simulink model "SCo1"  (Simulink 8.5)
settings: Solver=ode23tb  SolverMode=SingleTasking  StartTime=0.0  StopTime=0.1  MaxStep=2e-4  RelTol=1e-3  AbsTol=1e-6
libraries: powerlib x81, powerlib_extras x30
settings Model: Creator=azadpour  LastModifiedBy=PC  ExtModeTrigMode=oneshot  ExtModeArmWhenConnect=off
settings DataIOCC: LimitDataPoints=off
settings OptimizationCC: BlockReduction=off  BooleanDataType=off  InitFltsAndDblsToZero=on
settings DebuggingCC: SaveWithParameterizedLinksMsg=none  SignalResolutionControl=TryResolveAllWithWarning  MultiTaskDSMMsg=warning  MultiTaskCondExecSysMsg=none  FcnCallInpInsideContextMsg=UseLocalSettings
settings HardwareCC: TargetUnknown=on
settings GRTTargetCC: TargetFcnLib=ansi_tfl_tmw.mat

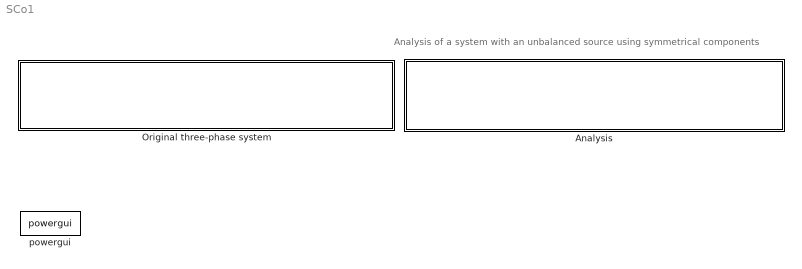
== system SCo1 ==
  note: Analysis of a system with an unbalanced source using symmetrical components
  Analysis : Subsystem
      mask Display: disp('Analysis of the system using Symmetrical Networks');
  Original three-phase system : Subsystem  mask(Original Three-phase system with unbalanced source){}
      mask Display: disp('Original Three-phase system with unbalanced source')
  powergui : powerlib/powergui  SimulationMode=Continuous  SolverType=Tustin/Backward Euler (TBE)  SampleTime=0  frequency=60  SPID=off  DisableSnubberDevices=off  DisableRonSwitches=off  DisableVfSwitches=off  SwTol=0  DisplayEquations=off  Interpol=off  methode=off  Ts=0  FunctionMessages=off  echomessages=off  HookPort=off  EnableUseOfTLC=off  x0status=blocks  frequencyindice=60  Pbase=100e6  ErrMax=1e-4  Iterations=50  UnitsV=kV  UnitsW=MW  buscounter=0  RestoreLinks=warning  ResistiveCurrentMeasurement=off  Frange=[0:2:500]  Ylog=off  Xlog=on  ShowGrid=off  save=off  variable=ZData  structure=0  ZoomFFT=on  StartTime=0.0  cycles=1  DisplayStyle=1  fundamental=60  FreqAxis=off  MaxFrequency=1000  frequencyindicesteady=1  RmsSteady=1  display=off

== system SCo1/Analysis ==
  note: Analysis using symmetrical networks
  Connected Sequence Networks : Subsystem
      mask Display: disp('Connected\n Sequence\n Networks')
  Negative Sequence Network : Subsystem
      mask Display: disp('Negative sequence network')
  Network with source decomposed in  symmetrical components : Subsystem
      mask Display: disp('Network with \nsource decomposed in\n symmetrical components')
  Positive Sequence Network : Subsystem
      mask Display: disp('Positive sequence network')
  Zero Sequence Network : Subsystem
      mask Display: disp('Zero sequence network')

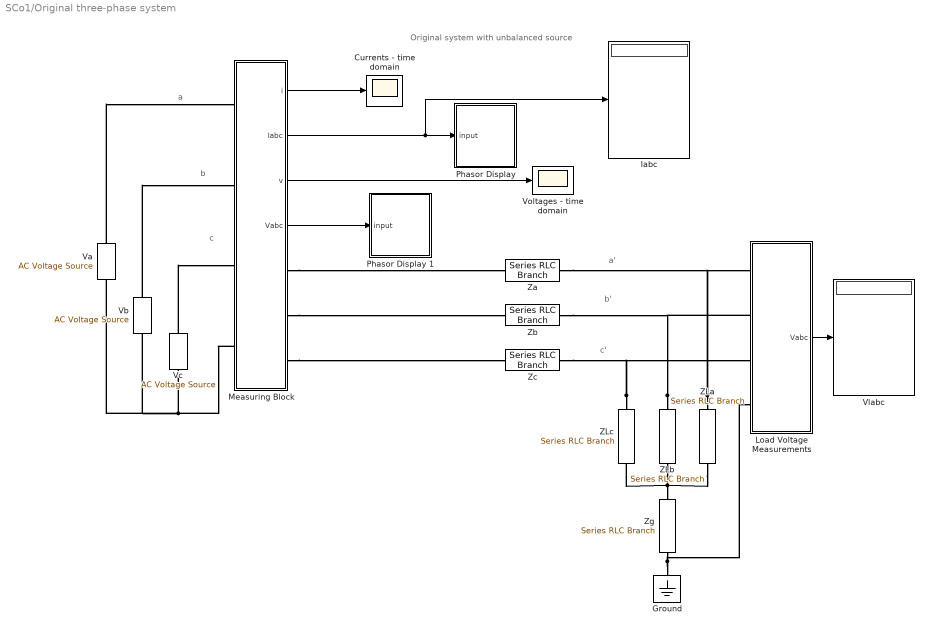
== system SCo1/Original three-phase system ==
  note: a
  note: a'
  note: b
  note: b'
  note: c'
  note: c
  note: Original system with unbalanced source
  Currents - time domain : Scope
      settings: TickLabels=on
  Ground : powerlib/Elements/Ground  LConnTagsString=a
  Iabc : Display
  Load Voltage Measurements : Subsystem
  Measuring Block : Subsystem
  Phasor Display : Subsystem  mask(ABC and 012 Phasor Display){Bactive=off}
      mask prompts: Bactive "Block active"
      mask init:
      | global count;
      | count=0;
      mask Help: web(['file:///' which('uc.html')]);
      mask Display: disp('Display \nabc \nand \n012\nphasors');
  Phasor Display 1 : Subsystem  mask(ABC and 012 Phasor Display){Bactive=off}
      mask prompts: Bactive "Block active"
      mask init:
      | global count;
      | count=0;
      mask Help: web(['file:///' which('uc.html')]);
      mask Display: disp('Display \nabc \nand \n012\nphasors');
  Va : powerlib/Electrical Sources/AC Voltage Source  Amplitude=1  Phase=0  Frequency=60  SampleTime=0  Measurements=None
  Vb : powerlib/Electrical Sources/AC Voltage Source  Amplitude=0.8  Phase=-110  Frequency=60  SampleTime=0  Measurements=None
  Vc : powerlib/Electrical Sources/AC Voltage Source  Amplitude=1.1  Phase=160  Frequency=60  SampleTime=0  Measurements=None
  Vlabc : Display
  Voltages - time domain : Scope
      settings: TickLabels=on
  ZLa : powerlib/Elements/Series RLC Branch  LConnTagsString=__new0  RConnTagsString=__new0  BranchType=RL  Resistance=0.1736  Inductance=0.9848/(2*pi*60)  SetiL0=off  InitialCurrent=0  Capacitance=1.0  Setx0=off  InitialVoltage=0  Measurements=None
  ZLb : powerlib/Elements/Series RLC Branch  LConnTagsString=__new0  RConnTagsString=__new0  BranchType=RL  Resistance=0.1736  Inductance=0.9848/(2*pi*60)  SetiL0=off  InitialCurrent=0  Capacitance=1.0  Setx0=off  InitialVoltage=0  Measurements=None
  ZLc : powerlib/Elements/Series RLC Branch  LConnTagsString=__new0  RConnTagsString=__new0  BranchType=RL  Resistance=0.1736  Inductance=0.9848/(2*pi*60)  SetiL0=off  InitialCurrent=0  Capacitance=1.0  Setx0=off  InitialVoltage=0  Measurements=None
  Za : powerlib/Elements/Series RLC Branch  LConnTagsString=__new0  RConnTagsString=__new0  BranchType=RL  Resistance=0.0347  Inductance=0.1970/(2*pi*60)  SetiL0=off  InitialCurrent=0  Capacitance=1.0  Setx0=off  InitialVoltage=0  Measurements=None
  Zb : powerlib/Elements/Series RLC Branch  LConnTagsString=__new0  RConnTagsString=__new0  BranchType=RL  Resistance=0.0347  Inductance=0.1970/(2*pi*60)  SetiL0=off  InitialCurrent=0  Capacitance=1.0  Setx0=off  InitialVoltage=0  Measurements=None
  Zc : powerlib/Elements/Series RLC Branch  LConnTagsString=__new0  RConnTagsString=__new0  BranchType=RL  Resistance=0.0347  Inductance=0.1970/(2*pi*60)  SetiL0=off  InitialCurrent=0  Capacitance=1.0  Setx0=off  InitialVoltage=0  Measurements=None
  Zg : powerlib/Elements/Series RLC Branch  LConnTagsString=__new0  RConnTagsString=__new0  BranchType=RL  Resistance=0.0695  Inductance=0.3939/(2*pi*60)  SetiL0=off  InitialCurrent=0  Capacitance=1.0  Setx0=off  InitialVoltage=0  Measurements=None
  wires:
  Measuring Block/1(i) -> Currents - time domain/1
  Measuring Block/3(v) -> Voltages - time domain/1
  Measuring Block/4(Vabc) -> Phasor Display 1/1(input)
  Load Voltage Measurements/1(Vabc) -> Vlabc/1
  Measuring Block/2(Iabc) -> Phasor Display/1(input), Iabc/1
  connections:
  Measuring Block/RConn1 -- Za/LConn1
  Measuring Block/RConn2 -- Zb/LConn1
  Measuring Block/RConn3 -- Zc/LConn1
  Va/LConn1 -- Vb/LConn1 -- Measuring Block/LConn4 -- Vc/LConn1
  Va/RConn1 -- Measuring Block/LConn1
  Vb/RConn1 -- Measuring Block/LConn2
  Vc/RConn1 -- Measuring Block/LConn3
  ZLb/RConn1 -- ZLa/RConn1 -- ZLc/RConn1 -- Zg/LConn1
  ZLb/LConn1 -- Load Voltage Measurements/LConn2 -- Zb/RConn1
  Ground/LConn1 -- Load Voltage Measurements/LConn4 -- Zg/RConn1
  ZLc/LConn1 -- Zc/RConn1 -- Load Voltage Measurements/LConn3
  ZLa/LConn1 -- Za/RConn1 -- Load Voltage Measurements/LConn1

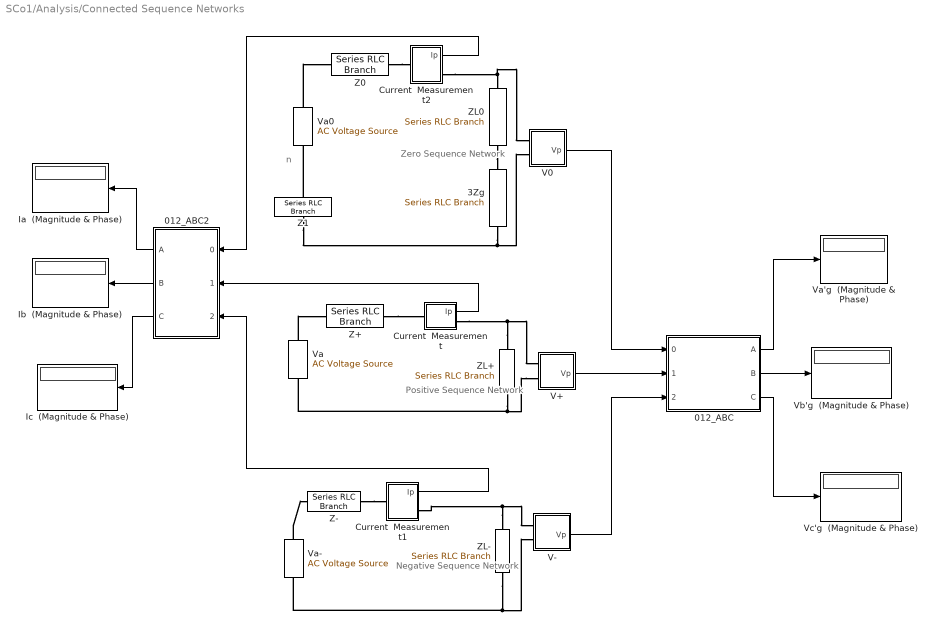
== system SCo1/Analysis/Connected Sequence Networks ==
  note: Positive Sequence Network
  note: Negative Sequence Network
  note: Zero Sequence Network
  note: n
  012_ABC : Subsystem
      mask init:
      | a=cos(120*pi/180)+i*sin(120*pi/180);
      | A=[1 1 1; 1 a^2 a; 1 a a^2];
      mask Display: disp('012_ABC');
  012_ABC2 : Subsystem
      mask init:
      | a=cos(120*pi/180)+i*sin(120*pi/180);
      | A=[1 1 1; 1 a^2 a; 1 a a^2];
      mask Display: disp('012_ABC');
  3Zg : powerlib/Elements/Series RLC Branch  LConnTagsString=__new0  RConnTagsString=__new0  BranchType=RL  Resistance=3*0.0695  Inductance=3*0.3939/(2*pi*60)  SetiL0=off  InitialCurrent=0  Capacitance=1.0  Setx0=off  InitialVoltage=0  Measurements=None
  Current  Measurement : Subsystem
  Current  Measurement1 : Subsystem
  Current  Measurement2 : Subsystem
  Ia  (Magnitude & Phase) : Display
  Ib  (Magnitude & Phase) : Display
  Ic  (Magnitude & Phase) : Display
  V+ : Subsystem
  V- : Subsystem
  V0 : Subsystem
  Va : powerlib/Electrical Sources/AC Voltage Source  Amplitude=0.92  Phase=17.8  Frequency=60  SampleTime=0  Measurements=None
  Va'g  (Magnitude & Phase) : Display
  Va- : powerlib/Electrical Sources/AC Voltage Source  Amplitude=0.27  Phase=-34.8  Frequency=60  SampleTime=0  Measurements=None
  Va0 : powerlib/Electrical Sources/AC Voltage Source  Amplitude=0.16  Phase=-129.3  Frequency=60  SampleTime=0  Measurements=None
  Vb'g  (Magnitude & Phase) : Display
  Vc'g  (Magnitude & Phase) : Display
  Z+ : powerlib/Elements/Series RLC Branch  LConnTagsString=__new0  RConnTagsString=__new0  BranchType=RL  Resistance=0.0347  Inductance=0.1970/(2*pi*60)  SetiL0=off  InitialCurrent=0  Capacitance=1.0  Setx0=off  InitialVoltage=0  Measurements=None
  Z- : powerlib/Elements/Series RLC Branch  LConnTagsString=__new0  RConnTagsString=__new0  BranchType=RL  Resistance=0.0347  Inductance=0.1970/(2*pi*60)  SetiL0=off  InitialCurrent=0  Capacitance=1.0  Setx0=off  InitialVoltage=0  Measurements=None
  Z0 : powerlib/Elements/Series RLC Branch  LConnTagsString=__new0  RConnTagsString=__new0  BranchType=RL  Resistance=0.0347  Inductance=0.1970/(2*pi*60)  SetiL0=off  InitialCurrent=0  Capacitance=1.0  Setx0=off  InitialVoltage=0  Measurements=None
  Z1 : powerlib/Elements/Series RLC Branch  LConnTagsString=__new0  RConnTagsString=__new0  BranchType=R  Resistance=1e10  Inductance=1.0  SetiL0=off  InitialCurrent=0  Capacitance=1.0  Setx0=off  InitialVoltage=0  Measurements=None
  ZL+ : powerlib/Elements/Series RLC Branch  LConnTagsString=__new0  RConnTagsString=__new0  BranchType=RL  Resistance=0.1736  Inductance=0.9848/(2*pi*60)  SetiL0=off  InitialCurrent=0  Capacitance=1.0  Setx0=off  InitialVoltage=0  Measurements=None
  ZL- : powerlib/Elements/Series RLC Branch  LConnTagsString=__new0  RConnTagsString=__new0  BranchType=RL  Resistance=0.1736  Inductance=0.9848/(2*pi*60)  SetiL0=off  InitialCurrent=0  Capacitance=1.0  Setx0=off  InitialVoltage=0  Measurements=None
  ZL0 : powerlib/Elements/Series RLC Branch  LConnTagsString=__new0  RConnTagsString=__new0  BranchType=RL  Resistance=0.1736  Inductance=0.9848/(2*pi*60)  SetiL0=off  InitialCurrent=0  Capacitance=1.0  Setx0=off  InitialVoltage=0  Measurements=None
  wires:
  012_ABC/1(A) -> Va'g  (Magnitude & Phase)/1
  012_ABC/2(B) -> Vb'g  (Magnitude & Phase)/1
  012_ABC/3(C) -> Vc'g  (Magnitude & Phase)/1
  012_ABC2/1(A) -> Ia  (Magnitude & Phase)/1
  012_ABC2/2(B) -> Ib  (Magnitude & Phase)/1
  012_ABC2/3(C) -> Ic  (Magnitude & Phase)/1
  Current  Measurement/1(Ip) -> 012_ABC2/2(1)
  V+/1(Vp) -> 012_ABC/2(1)
  V-/1(Vp) -> 012_ABC/3(2)
  Current  Measurement1/1(Ip) -> 012_ABC2/3(2)
  V0/1(Vp) -> 012_ABC/1(0)
  Current  Measurement2/1(Ip) -> 012_ABC2/1(0)
  connections:
  V+/LConn2 -- Va/LConn1 -- ZL+/RConn1
  ZL+/LConn1 -- Current  Measurement/RConn1 -- V+/LConn1
  Va-/LConn1 -- ZL-/RConn1 -- V-/LConn2
  ZL-/LConn1 -- Current  Measurement1/RConn1 -- V-/LConn1
  ZL0/LConn1 -- Current  Measurement2/RConn1 -- V0/LConn1
  3Zg/RConn1 -- Z1/LConn1 -- V0/LConn2
  Z+/RConn1 -- Current  Measurement/LConn1
  Z-/RConn1 -- Current  Measurement1/LConn1
  Va-/RConn1 -- Z-/LConn1
  Z0/RConn1 -- Current  Measurement2/LConn1
  Z1/RConn1 -- Va0/LConn1
  Va0/RConn1 -- Z0/LConn1
  Va/RConn1 -- Z+/LConn1
  ZL0/RConn1 -- 3Zg/LConn1

== system SCo1/Analysis/Negative Sequence Network ==
  Current  Measurement : Subsystem
  "Ia- (Magnitude & Phase) " : Display
  V- : Subsystem
  Va'g- (Magnitude & Phase) : Display
  Va- : powerlib/Electrical Sources/AC Voltage Source  Amplitude=0.27  Phase=-34.8  Frequency=60  SampleTime=0  Measurements=None
  ZLa : powerlib/Elements/Series RLC Branch  LConnTagsString=__new0  RConnTagsString=__new0  BranchType=RL  Resistance=0.1736  Inductance=0.9848/(2*pi*60)  SetiL0=off  InitialCurrent=0  Capacitance=1.0  Setx0=off  InitialVoltage=0  Measurements=None
  Za : powerlib/Elements/Series RLC Branch  LConnTagsString=__new0  RConnTagsString=__new0  BranchType=RL  Resistance=0.0347  Inductance=0.1970/(2*pi*60)  SetiL0=off  InitialCurrent=0  Capacitance=1.0  Setx0=off  InitialVoltage=0  Measurements=None
  wires:
  Current  Measurement/1(Ip) -> "Ia- (Magnitude & Phase) "/1
  V-/1(V) -> Va'g- (Magnitude & Phase)/1
  connections:
  Va-/RConn1 -- Za/LConn1
  ZLa/RConn1 -- V-/LConn2 -- Va-/LConn1
  Za/RConn1 -- Current  Measurement/LConn1
  Current  Measurement/RConn1 -- V-/LConn1 -- ZLa/LConn1

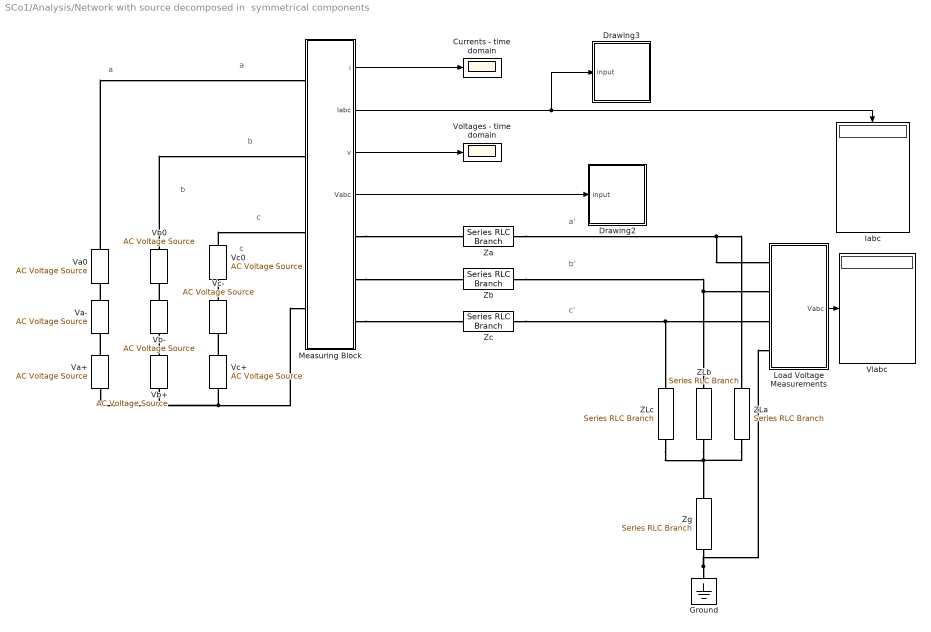
== system SCo1/Analysis/Network with source decomposed in  symmetrical components ==
  note: a
  note: b
  note: a
  note: a'
  note: b
  note: b'
  note: c'
  note: c
  note: c
  Currents - time domain : Scope
      settings: TickLabels=on
  Drawing2 : Subsystem  mask(ABC and 012 Phasor Display){Bactive=off}
      mask prompts: Bactive "Block active"
      mask init:
      | global count;
      | count=0;
      mask Help: web(['file:///' which('uc.html')]);
      mask Display: disp('Display \nabc \nand \n012\nphasors');
  Drawing3 : Subsystem  mask(ABC and 012 Phasor Display){Bactive=off}
      mask prompts: Bactive "Block active"
      mask init:
      | global count;
      | count=0;
      mask Help: web(['file:///' which('uc.html')]);
      mask Display: disp('Display \nabc \nand \n012\nphasors');
  Ground : powerlib/Elements/Ground  LConnTagsString=a
  Iabc : Display
  Load Voltage Measurements : Subsystem
  Measuring Block : Subsystem
  Va+ : powerlib/Electrical Sources/AC Voltage Source  Amplitude=0.92  Phase=17.8  Frequency=60  SampleTime=0  Measurements=None
  Va- : powerlib/Electrical Sources/AC Voltage Source  Amplitude=0.27  Phase=-34.8  Frequency=60  SampleTime=0  Measurements=None
  Va0 : powerlib/Electrical Sources/AC Voltage Source  Amplitude=0.16  Phase=-129.3  Frequency=60  SampleTime=0  Measurements=None
  Vb+ : powerlib/Electrical Sources/AC Voltage Source  Amplitude=0.92  Phase=17.8-120  Frequency=60  SampleTime=0  Measurements=None
  Vb- : powerlib/Electrical Sources/AC Voltage Source  Amplitude=0.27  Phase=-34.8+120  Frequency=60  SampleTime=0  Measurements=None
  Vb0 : powerlib/Electrical Sources/AC Voltage Source  Amplitude=0.16  Phase=-129.3  Frequency=60  SampleTime=0  Measurements=None
  Vc+ : powerlib/Electrical Sources/AC Voltage Source  Amplitude=0.92  Phase=17.8+120  Frequency=60  SampleTime=0  Measurements=None
  Vc- : powerlib/Electrical Sources/AC Voltage Source  Amplitude=0.27  Phase=-34.8-120  Frequency=60  SampleTime=0  Measurements=None
  Vc0 : powerlib/Electrical Sources/AC Voltage Source  Amplitude=0.16  Phase=-129.3  Frequency=60  SampleTime=0  Measurements=None
  Vlabc : Display
  Voltages - time domain : Scope
      settings: TickLabels=on
  ZLa : powerlib/Elements/Series RLC Branch  LConnTagsString=__new0  RConnTagsString=__new0  BranchType=RL  Resistance=0.1736  Inductance=0.9848/(2*pi*60)  SetiL0=off  InitialCurrent=0  Capacitance=1.0  Setx0=off  InitialVoltage=0  Measurements=None
  ZLb : powerlib/Elements/Series RLC Branch  LConnTagsString=__new0  RConnTagsString=__new0  BranchType=RL  Resistance=0.1736  Inductance=0.9848/(2*pi*60)  SetiL0=off  InitialCurrent=0  Capacitance=1.0  Setx0=off  InitialVoltage=0  Measurements=None
  ZLc : powerlib/Elements/Series RLC Branch  LConnTagsString=__new0  RConnTagsString=__new0  BranchType=RL  Resistance=0.1736  Inductance=0.9848/(2*pi*60)  SetiL0=off  InitialCurrent=0  Capacitance=1.0  Setx0=off  InitialVoltage=0  Measurements=None
  Za : powerlib/Elements/Series RLC Branch  LConnTagsString=__new0  RConnTagsString=__new0  BranchType=RL  Resistance=0.0347  Inductance=0.1970/(2*pi*60)  SetiL0=off  InitialCurrent=0  Capacitance=1.0  Setx0=off  InitialVoltage=0  Measurements=None
  Zb : powerlib/Elements/Series RLC Branch  LConnTagsString=__new0  RConnTagsString=__new0  BranchType=RL  Resistance=0.0347  Inductance=0.1970/(2*pi*60)  SetiL0=off  InitialCurrent=0  Capacitance=1.0  Setx0=off  InitialVoltage=0  Measurements=None
  Zc : powerlib/Elements/Series RLC Branch  LConnTagsString=__new0  RConnTagsString=__new0  BranchType=RL  Resistance=0.0347  Inductance=0.1970/(2*pi*60)  SetiL0=off  InitialCurrent=0  Capacitance=1.0  Setx0=off  InitialVoltage=0  Measurements=None
  Zg : powerlib/Elements/Series RLC Branch  LConnTagsString=__new0  RConnTagsString=__new0  BranchType=RL  Resistance=0.0695  Inductance=0.3939/(2*pi*60)  SetiL0=off  InitialCurrent=0  Capacitance=1.0  Setx0=off  InitialVoltage=0  Measurements=None
  wires:
  Load Voltage Measurements/1(Vabc) -> Vlabc/1
  Measuring Block/1(i) -> Currents - time domain/1
  Measuring Block/3(v) -> Voltages - time domain/1
  Measuring Block/4(Vabc) -> Drawing2/1(input)
  Measuring Block/2(Iabc) -> Iabc/1, Drawing3/1(input)
  connections:
  Measuring Block/RConn1 -- Za/LConn1
  Measuring Block/RConn2 -- Zb/LConn1
  Measuring Block/RConn3 -- Zc/LConn1
  Vb0/RConn1 -- Measuring Block/LConn2
  Va0/RConn1 -- Measuring Block/LConn1
  Vc0/RConn1 -- Measuring Block/LConn3
  Va-/RConn1 -- Va0/LConn1
  Ground/LConn1 -- Load Voltage Measurements/LConn4 -- Zg/RConn1
  Zc/RConn1 -- ZLc/LConn1 -- Load Voltage Measurements/LConn3
  Zb/RConn1 -- ZLb/LConn1 -- Load Voltage Measurements/LConn2
  Za/RConn1 -- ZLa/LConn1 -- Load Voltage Measurements/LConn1
  Va+/RConn1 -- Va-/LConn1
  Vb+/RConn1 -- Vb-/LConn1
  Vc+/RConn1 -- Vc-/LConn1
  Vc-/RConn1 -- Vc0/LConn1
  Vb-/RConn1 -- Vb0/LConn1
  Va+/LConn1 -- Vb+/LConn1 -- Measuring Block/LConn4 -- Vc+/LConn1
  ZLb/RConn1 -- Zg/LConn1 -- ZLa/RConn1 -- ZLc/RConn1

== system SCo1/Analysis/Positive Sequence Network ==
  Current  Measurement : Subsystem
  Ia+ (Magnitude & Phase)1 : Display
  V+ : Subsystem
  Va'g+ (Magnitude & Phase) : Display
  Va+ : powerlib/Electrical Sources/AC Voltage Source  Amplitude=0.92  Phase=17.8  Frequency=60  SampleTime=0  Measurements=None
  ZLa : powerlib/Elements/Series RLC Branch  LConnTagsString=__new0  RConnTagsString=__new0  BranchType=RL  Resistance=0.1736  Inductance=0.9848/(2*pi*60)  SetiL0=off  InitialCurrent=0  Capacitance=1.0  Setx0=off  InitialVoltage=0  Measurements=None
  Za : powerlib/Elements/Series RLC Branch  LConnTagsString=__new0  RConnTagsString=__new0  BranchType=RL  Resistance=0.0347  Inductance=0.1970/(2*pi*60)  SetiL0=off  InitialCurrent=0  Capacitance=1.0  Setx0=off  InitialVoltage=0  Measurements=None
  wires:
  V+/1(V) -> Va'g+ (Magnitude & Phase)/1
  Current  Measurement/1(Ip) -> Ia+ (Magnitude & Phase)1/1
  connections:
  Va+/RConn1 -- Za/LConn1
  ZLa/RConn1 -- V+/LConn2 -- Va+/LConn1
  Za/RConn1 -- Current  Measurement/LConn1
  Current  Measurement/RConn1 -- ZLa/LConn1 -- V+/LConn1

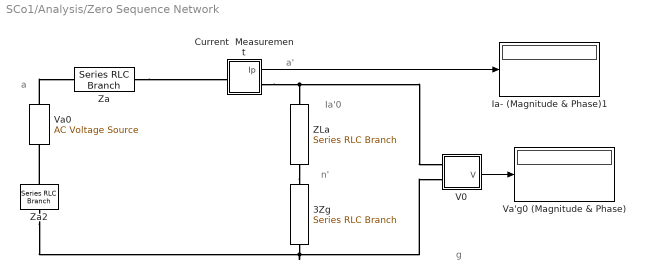
== system SCo1/Analysis/Zero Sequence Network ==
  note: n'
  note: a
  note: a'
  note: g
  note: Ia'0
  3Zg : powerlib/Elements/Series RLC Branch  LConnTagsString=__new0  RConnTagsString=__new0  BranchType=RL  Resistance=3*0.0695  Inductance=3*0.3939/(2*pi*60)  SetiL0=off  InitialCurrent=0  Capacitance=1.0  Setx0=off  InitialVoltage=0  Measurements=None
  Current  Measurement : Subsystem
  Ia- (Magnitude & Phase)1 : Display
      settings: Decimation=2
  V0 : Subsystem
  Va'g0 (Magnitude & Phase) : Display
  Va0 : powerlib/Electrical Sources/AC Voltage Source  Amplitude=0.16  Phase=-129.3  Frequency=60  SampleTime=0  Measurements=None
  ZLa : powerlib/Elements/Series RLC Branch  LConnTagsString=__new0  RConnTagsString=__new0  BranchType=RL  Resistance=0.1736  Inductance=0.9848/(2*pi*60)  SetiL0=off  InitialCurrent=0  Capacitance=1.0  Setx0=off  InitialVoltage=0  Measurements=None
  Za : powerlib/Elements/Series RLC Branch  LConnTagsString=__new0  RConnTagsString=__new0  BranchType=RL  Resistance=0.0347  Inductance=0.1970/(2*pi*60)  SetiL0=off  InitialCurrent=0  Capacitance=1.0  Setx0=off  InitialVoltage=0  Measurements=None
  Za2 : powerlib/Elements/Series RLC Branch  LConnTagsString=__new0  RConnTagsString=__new0  BranchType=Open circuit  Resistance=1  Inductance=1e-3  SetiL0=off  InitialCurrent=0  Capacitance=1e-6  Setx0=off  InitialVoltage=0  Measurements=None
  wires:
  V0/1(V) -> Va'g0 (Magnitude & Phase)/1
  Current  Measurement/1(Ip) -> Ia- (Magnitude & Phase)1/1
  connections:
  ZLa/RConn1 -- 3Zg/LConn1
  Va0/RConn1 -- Za/LConn1
  Za/RConn1 -- Current  Measurement/LConn1
  Za2/RConn1 -- 3Zg/RConn1 -- V0/LConn2
  Current  Measurement/RConn1 -- V0/LConn1 -- ZLa/LConn1
  Za2/LConn1 -- Va0/LConn1

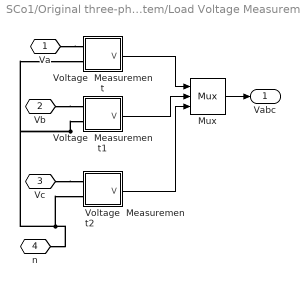
== system SCo1/Original three-phase system/Load Voltage Measurements ==
  Mux : Mux  Inputs=3
  Voltage  Measurement : Subsystem
  Voltage  Measurement1 : Subsystem
  Voltage  Measurement2 : Subsystem
  Va : PMIOPort  Port=1  Side=Left
  Vb : PMIOPort  Port=2  Side=Left
  Vc : PMIOPort  Port=3  Side=Left
  n : PMIOPort  Port=4  Side=Left
  Vabc : Outport  InitialOutput=0
  wires:
  Voltage  Measurement/1(V) -> Mux/1
  Voltage  Measurement1/1(V) -> Mux/2
  Voltage  Measurement2/1(V) -> Mux/3
  Mux/1 -> Vabc/1
  connections:
  Va/RConn1 -- Voltage  Measurement/LConn1
  Vb/RConn1 -- Voltage  Measurement1/LConn1
  Vc/RConn1 -- Voltage  Measurement2/LConn1
  n/RConn1 -- Voltage  Measurement2/LConn2 -- Voltage  Measurement1/LConn2 -- Voltage  Measurement/LConn2

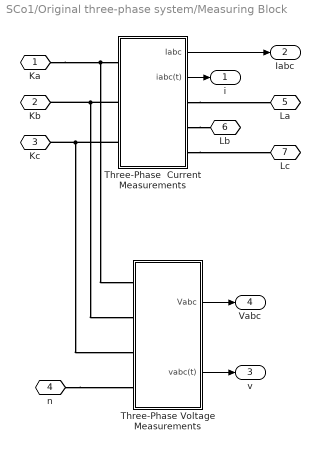
== system SCo1/Original three-phase system/Measuring Block ==
  Three-Phase Voltage Measurements : Subsystem
  Three-Phase  Current Measurements : Subsystem
  Ka : PMIOPort  Port=1  Side=Left
  Kb : PMIOPort  Port=2  Side=Left
  Kc : PMIOPort  Port=3  Side=Left
  n : PMIOPort  Port=4  Side=Left
  La : PMIOPort  Port=5  Side=Right
  Lb : PMIOPort  Port=6  Side=Right
  Lc : PMIOPort  Port=7  Side=Right
  i : Outport
  Iabc : Outport  Port=2
  v : Outport  Port=3
  Vabc : Outport  Port=4
  wires:
  Three-Phase  Current Measurements/1(Iabc) -> Iabc/1
  Three-Phase Voltage Measurements/1(Vabc) -> Vabc/1
  Three-Phase  Current Measurements/2(iabc(t)) -> i/1
  Three-Phase Voltage Measurements/2(vabc(t)) -> v/1
  connections:
  Three-Phase  Current Measurements/RConn3 -- Lc/RConn1
  Three-Phase  Current Measurements/RConn2 -- Lb/RConn1
  Three-Phase  Current Measurements/RConn1 -- La/RConn1
  n/RConn1 -- Three-Phase Voltage Measurements/LConn4
  Ka/RConn1 -- Three-Phase  Current Measurements/LConn1 -- Three-Phase Voltage Measurements/LConn1
  Three-Phase  Current Measurements/LConn2 -- Kb/RConn1 -- Three-Phase Voltage Measurements/LConn2
  Three-Phase  Current Measurements/LConn3 -- Kc/RConn1 -- Three-Phase Voltage Measurements/LConn3

== system SCo1/Original three-phase system/Phasor Display ==
  input : Inport
  S-Function : S-Function  FunctionName=phdraw1c  Parameters=Bactive
  wires:
  input/1 -> S-Function/1

== system SCo1/Original three-phase system/Phasor Display 1 ==
  input : Inport
  S-Function : S-Function  FunctionName=phdraw1c  Parameters=Bactive
  wires:
  input/1 -> S-Function/1

== system SCo1/Analysis/Connected Sequence Networks/012_ABC ==
  0 : Inport
  1 : Inport  Port=2
  2 : Inport  Port=3
  Demux : Demux  Outputs=3
  Mux3 : Mux  Inputs=3
  S-Function : S-Function  FunctionName=pnz_ABC  Parameters=A
  A : Outport  InitialOutput=0
  B : Outport  Port=2  InitialOutput=0
  C : Outport  Port=3  InitialOutput=0
  wires:
  Mux3/1 -> S-Function/1
  0/1 -> Mux3/1
  1/1 -> Mux3/2
  2/1 -> Mux3/3
  S-Function/1 -> Demux/1
  Demux/1 -> A/1
  Demux/2 -> B/1
  Demux/3 -> C/1

== system SCo1/Analysis/Connected Sequence Networks/012_ABC2 ==
  0 : Inport
  1 : Inport  Port=2
  2 : Inport  Port=3
  Demux : Demux  Outputs=3
  Mux3 : Mux  Inputs=3
  S-Function : S-Function  FunctionName=pnz_ABC  Parameters=A
  A : Outport  InitialOutput=0
  B : Outport  Port=2  InitialOutput=0
  C : Outport  Port=3  InitialOutput=0
  wires:
  Demux/3 -> C/1
  Demux/2 -> B/1
  Demux/1 -> A/1
  S-Function/1 -> Demux/1
  2/1 -> Mux3/3
  1/1 -> Mux3/2
  0/1 -> Mux3/1
  Mux3/1 -> S-Function/1

== system SCo1/Analysis/Connected Sequence Networks/Current  Measurement ==
  Current Measurement1 : powerlib/Measurements/Current Measurement  PhasorSimulation=off  OutputType=Magnitude  PSBequivalent=0
  Fourier1 : powerlib_extras/Measurements/Fourier  f1=60  n=1
  Mux1 : Mux  Inputs=2
  + : PMIOPort  Port=1  Side=Left
  - : PMIOPort  Port=2  Side=Right
  Ip : Outport  InitialOutput=0
  wires:
  Fourier1/2 -> Mux1/2
  Fourier1/1 -> Mux1/1
  Mux1/1 -> Ip/1
  Current Measurement1/1 -> Fourier1/1
  connections:
  +/RConn1 -- Current Measurement1/LConn1
  Current Measurement1/RConn1 -- -/RConn1

== system SCo1/Analysis/Connected Sequence Networks/Current  Measurement1 ==
  Current Measurement1 : powerlib/Measurements/Current Measurement  PhasorSimulation=off  OutputType=Magnitude  PSBequivalent=0
  Fourier1 : powerlib_extras/Measurements/Fourier  f1=60  n=1
  Mux1 : Mux  Inputs=2
  + : PMIOPort  Port=1  Side=Left
  - : PMIOPort  Port=2  Side=Right
  Ip : Outport  InitialOutput=0
  wires:
  Fourier1/2 -> Mux1/2
  Fourier1/1 -> Mux1/1
  Mux1/1 -> Ip/1
  Current Measurement1/1 -> Fourier1/1
  connections:
  +/RConn1 -- Current Measurement1/LConn1
  Current Measurement1/RConn1 -- -/RConn1

== system SCo1/Analysis/Connected Sequence Networks/Current  Measurement2 ==
  Current Measurement1 : powerlib/Measurements/Current Measurement  PhasorSimulation=off  OutputType=Magnitude  PSBequivalent=0
  Fourier1 : powerlib_extras/Measurements/Fourier  f1=60  n=1
  Mux1 : Mux  Inputs=2
  + : PMIOPort  Port=1  Side=Left
  - : PMIOPort  Port=2  Side=Right
  Ip : Outport  InitialOutput=0
  wires:
  Fourier1/2 -> Mux1/2
  Fourier1/1 -> Mux1/1
  Mux1/1 -> Ip/1
  Current Measurement1/1 -> Fourier1/1
  connections:
  +/RConn1 -- Current Measurement1/LConn1
  Current Measurement1/RConn1 -- -/RConn1

== system SCo1/Analysis/Connected Sequence Networks/V+ ==
  Fourier2 : powerlib_extras/Measurements/Fourier  f1=60  n=1
  Mux3 : Mux  Inputs=2
  Voltage Measurement1 : powerlib/Measurements/Voltage Measurement  PhasorSimulation=off  OutputType=Magnitude  PSBequivalent=0
  + : PMIOPort  Port=1  Side=Left
  - : PMIOPort  Port=2  Side=Left
  Vp : Outport  InitialOutput=0
  wires:
  Fourier2/1 -> Mux3/1
  Fourier2/2 -> Mux3/2
  Mux3/1 -> Vp/1
  Voltage Measurement1/1 -> Fourier2/1
  connections:
  +/RConn1 -- Voltage Measurement1/LConn1
  -/RConn1 -- Voltage Measurement1/LConn2

== system SCo1/Analysis/Connected Sequence Networks/V- ==
  Fourier2 : powerlib_extras/Measurements/Fourier  f1=60  n=1
  Mux3 : Mux  Inputs=2
  Voltage Measurement1 : powerlib/Measurements/Voltage Measurement  PhasorSimulation=off  OutputType=Magnitude  PSBequivalent=0
  + : PMIOPort  Port=1  Side=Left
  - : PMIOPort  Port=2  Side=Left
  Vp : Outport  InitialOutput=0
  wires:
  Fourier2/1 -> Mux3/1
  Fourier2/2 -> Mux3/2
  Mux3/1 -> Vp/1
  Voltage Measurement1/1 -> Fourier2/1
  connections:
  +/RConn1 -- Voltage Measurement1/LConn1
  -/RConn1 -- Voltage Measurement1/LConn2

== system SCo1/Analysis/Connected Sequence Networks/V0 ==
  Fourier2 : powerlib_extras/Measurements/Fourier  f1=60  n=1
  Mux3 : Mux  Inputs=2
  Voltage Measurement1 : powerlib/Measurements/Voltage Measurement  PhasorSimulation=off  OutputType=Magnitude  PSBequivalent=0
  + : PMIOPort  Port=1  Side=Left
  - : PMIOPort  Port=2  Side=Left
  Vp : Outport  InitialOutput=0
  wires:
  Mux3/1 -> Vp/1
  Fourier2/2 -> Mux3/2
  Fourier2/1 -> Mux3/1
  Voltage Measurement1/1 -> Fourier2/1
  connections:
  -/RConn1 -- Voltage Measurement1/LConn2
  +/RConn1 -- Voltage Measurement1/LConn1

== system SCo1/Analysis/Negative Sequence Network/Current  Measurement ==
  Current Measurement1 : powerlib/Measurements/Current Measurement  PhasorSimulation=off  OutputType=Magnitude  PSBequivalent=0
  Fourier1 : powerlib_extras/Measurements/Fourier  f1=60  n=1
  Mux : Mux  Inputs=2
  + : PMIOPort  Port=1  Side=Left
  - : PMIOPort  Port=2  Side=Right
  Ip : Outport  InitialOutput=0
  wires:
  Fourier1/2 -> Mux/2
  Fourier1/1 -> Mux/1
  Current Measurement1/1 -> Fourier1/1
  Mux/1 -> Ip/1
  connections:
  +/RConn1 -- Current Measurement1/LConn1
  Current Measurement1/RConn1 -- -/RConn1

== system SCo1/Analysis/Negative Sequence Network/V- ==
  Fourier2 : powerlib_extras/Measurements/Fourier  f1=60  n=1
  Mux3 : Mux  Inputs=2
  Voltage Measurement1 : powerlib/Measurements/Voltage Measurement  PhasorSimulation=off  OutputType=Magnitude  PSBequivalent=0
  + : PMIOPort  Port=1  Side=Left
  - : PMIOPort  Port=2  Side=Left
  V : Outport  InitialOutput=0
  wires:
  Fourier2/1 -> Mux3/1
  Fourier2/2 -> Mux3/2
  Mux3/1 -> V/1
  Voltage Measurement1/1 -> Fourier2/1
  connections:
  +/RConn1 -- Voltage Measurement1/LConn1
  -/RConn1 -- Voltage Measurement1/LConn2

== system SCo1/Analysis/Network with source decomposed in  symmetrical components/Drawing2 ==
  input : Inport
  S-Function : S-Function  FunctionName=phdraw1c  Parameters=Bactive
  wires:
  input/1 -> S-Function/1

== system SCo1/Analysis/Network with source decomposed in  symmetrical components/Drawing3 ==
  input : Inport
  S-Function : S-Function  FunctionName=phdraw1c  Parameters=Bactive
  wires:
  input/1 -> S-Function/1

== system SCo1/Analysis/Network with source decomposed in  symmetrical components/Load Voltage Measurements ==
  Mux : Mux  Inputs=3
  Voltage  Measurement : Subsystem
  Voltage  Measurement1 : Subsystem
  Voltage  Measurement2 : Subsystem
  Va : PMIOPort  Port=1  Side=Left
  Vb : PMIOPort  Port=2  Side=Left
  Vc : PMIOPort  Port=3  Side=Left
  n : PMIOPort  Port=4  Side=Left
  Vabc : Outport  InitialOutput=0
  wires:
  Voltage  Measurement/1(V) -> Mux/1
  Voltage  Measurement1/1(V) -> Mux/2
  Voltage  Measurement2/1(V) -> Mux/3
  Mux/1 -> Vabc/1
  connections:
  Va/RConn1 -- Voltage  Measurement/LConn1
  Vb/RConn1 -- Voltage  Measurement1/LConn1
  Vc/RConn1 -- Voltage  Measurement2/LConn1
  n/RConn1 -- Voltage  Measurement2/LConn2 -- Voltage  Measurement1/LConn2 -- Voltage  Measurement/LConn2

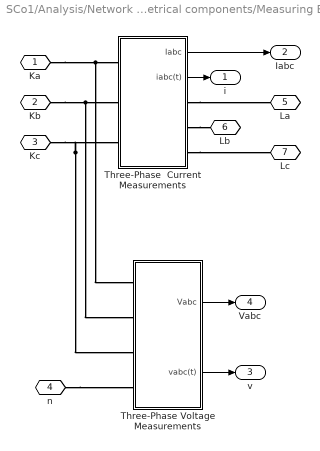
== system SCo1/Analysis/Network with source decomposed in  symmetrical components/Measuring Block ==
  Three-Phase Voltage Measurements : Subsystem
  Three-Phase  Current Measurements : Subsystem
  Ka : PMIOPort  Port=1  Side=Left
  Kb : PMIOPort  Port=2  Side=Left
  Kc : PMIOPort  Port=3  Side=Left
  n : PMIOPort  Port=4  Side=Left
  La : PMIOPort  Port=5  Side=Right
  Lb : PMIOPort  Port=6  Side=Right
  Lc : PMIOPort  Port=7  Side=Right
  i : Outport
  Iabc : Outport  Port=2
  v : Outport  Port=3
  Vabc : Outport  Port=4
  wires:
  Three-Phase  Current Measurements/1(Iabc) -> Iabc/1
  Three-Phase Voltage Measurements/1(Vabc) -> Vabc/1
  Three-Phase  Current Measurements/2(iabc(t)) -> i/1
  Three-Phase Voltage Measurements/2(vabc(t)) -> v/1
  connections:
  Three-Phase  Current Measurements/RConn3 -- Lc/RConn1
  Three-Phase  Current Measurements/RConn2 -- Lb/RConn1
  Three-Phase  Current Measurements/RConn1 -- La/RConn1
  n/RConn1 -- Three-Phase Voltage Measurements/LConn4
  Kc/RConn1 -- Three-Phase  Current Measurements/LConn3 -- Three-Phase Voltage Measurements/LConn3
  Ka/RConn1 -- Three-Phase  Current Measurements/LConn1 -- Three-Phase Voltage Measurements/LConn1
  Kb/RConn1 -- Three-Phase  Current Measurements/LConn2 -- Three-Phase Voltage Measurements/LConn2

== system SCo1/Analysis/Positive Sequence Network/Current  Measurement ==
  Current Measurement1 : powerlib/Measurements/Current Measurement  PhasorSimulation=off  OutputType=Magnitude  PSBequivalent=0
  Fourier1 : powerlib_extras/Measurements/Fourier  f1=60  n=1
  Mux1 : Mux  Inputs=2
  + : PMIOPort  Port=1  Side=Left
  - : PMIOPort  Port=2  Side=Right
  Ip : Outport  InitialOutput=0
  wires:
  Fourier1/2 -> Mux1/2
  Fourier1/1 -> Mux1/1
  Mux1/1 -> Ip/1
  Current Measurement1/1 -> Fourier1/1
  connections:
  +/RConn1 -- Current Measurement1/LConn1
  Current Measurement1/RConn1 -- -/RConn1

== system SCo1/Analysis/Positive Sequence Network/V+ ==
  Fourier2 : powerlib_extras/Measurements/Fourier  f1=60  n=1
  Mux3 : Mux  Inputs=2
  Voltage Measurement1 : powerlib/Measurements/Voltage Measurement  PhasorSimulation=off  OutputType=Magnitude  PSBequivalent=0
  + : PMIOPort  Port=1  Side=Left
  - : PMIOPort  Port=2  Side=Left
  V : Outport  InitialOutput=0
  wires:
  Fourier2/1 -> Mux3/1
  Fourier2/2 -> Mux3/2
  Mux3/1 -> V/1
  Voltage Measurement1/1 -> Fourier2/1
  connections:
  +/RConn1 -- Voltage Measurement1/LConn1
  -/RConn1 -- Voltage Measurement1/LConn2

== system SCo1/Analysis/Zero Sequence Network/Current  Measurement ==
  Current Measurement1 : powerlib/Measurements/Current Measurement  PhasorSimulation=off  OutputType=Magnitude  PSBequivalent=0
  Fourier1 : powerlib_extras/Measurements/Fourier  f1=60  n=1
  Mux1 : Mux  Inputs=2
  + : PMIOPort  Port=1  Side=Left
  - : PMIOPort  Port=2  Side=Right
  Ip : Outport  InitialOutput=0
  wires:
  Fourier1/2 -> Mux1/2
  Fourier1/1 -> Mux1/1
  Mux1/1 -> Ip/1
  Current Measurement1/1 -> Fourier1/1
  connections:
  +/RConn1 -- Current Measurement1/LConn1
  Current Measurement1/RConn1 -- -/RConn1

== system SCo1/Analysis/Zero Sequence Network/V0 ==
  Fourier2 : powerlib_extras/Measurements/Fourier  f1=60  n=1
  Mux3 : Mux  Inputs=2
  Voltage Measurement1 : powerlib/Measurements/Voltage Measurement  PhasorSimulation=off  OutputType=Magnitude  PSBequivalent=0
  + : PMIOPort  Port=1  Side=Left
  - : PMIOPort  Port=2  Side=Left
  V : Outport  InitialOutput=0
  wires:
  Fourier2/1 -> Mux3/1
  Fourier2/2 -> Mux3/2
  Mux3/1 -> V/1
  Voltage Measurement1/1 -> Fourier2/1
  connections:
  +/RConn1 -- Voltage Measurement1/LConn1
  -/RConn1 -- Voltage Measurement1/LConn2

== system SCo1/Original three-phase system/Load Voltage Measurements/Voltage  Measurement ==
  Fourier2 : powerlib_extras/Measurements/Fourier  f1=60  n=1
  Mux3 : Mux  Inputs=2
  Voltage Measurement1 : powerlib/Measurements/Voltage Measurement  PhasorSimulation=off  OutputType=Magnitude  PSBequivalent=0
  + : PMIOPort  Port=1  Side=Left
  - : PMIOPort  Port=2  Side=Left
  V : Outport  InitialOutput=0
  wires:
  Fourier2/1 -> Mux3/1
  Fourier2/2 -> Mux3/2
  Mux3/1 -> V/1
  Voltage Measurement1/1 -> Fourier2/1
  connections:
  +/RConn1 -- Voltage Measurement1/LConn1
  -/RConn1 -- Voltage Measurement1/LConn2

== system SCo1/Original three-phase system/Load Voltage Measurements/Voltage  Measurement1 ==
  Fourier2 : powerlib_extras/Measurements/Fourier  f1=60  n=1
  Mux3 : Mux  Inputs=2
  Voltage Measurement1 : powerlib/Measurements/Voltage Measurement  PhasorSimulation=off  OutputType=Magnitude  PSBequivalent=0
  + : PMIOPort  Port=1  Side=Left
  - : PMIOPort  Port=2  Side=Left
  V : Outport  InitialOutput=0
  wires:
  Mux3/1 -> V/1
  Fourier2/2 -> Mux3/2
  Fourier2/1 -> Mux3/1
  Voltage Measurement1/1 -> Fourier2/1
  connections:
  -/RConn1 -- Voltage Measurement1/LConn2
  +/RConn1 -- Voltage Measurement1/LConn1

== system SCo1/Original three-phase system/Load Voltage Measurements/Voltage  Measurement2 ==
  Fourier2 : powerlib_extras/Measurements/Fourier  f1=60  n=1
  Mux3 : Mux  Inputs=2
  Voltage Measurement1 : powerlib/Measurements/Voltage Measurement  PhasorSimulation=off  OutputType=Magnitude  PSBequivalent=0
  + : PMIOPort  Port=1  Side=Left
  - : PMIOPort  Port=2  Side=Left
  V : Outport  InitialOutput=0
  wires:
  Fourier2/1 -> Mux3/1
  Fourier2/2 -> Mux3/2
  Mux3/1 -> V/1
  Voltage Measurement1/1 -> Fourier2/1
  connections:
  +/RConn1 -- Voltage Measurement1/LConn1
  -/RConn1 -- Voltage Measurement1/LConn2

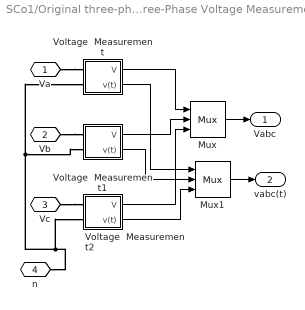
== system SCo1/Original three-phase system/Measuring Block/Three-Phase Voltage Measurements ==
  Mux : Mux  Inputs=3
  Mux1 : Mux  Inputs=3
  Voltage  Measurement : Subsystem
  Voltage  Measurement1 : Subsystem
  Voltage  Measurement2 : Subsystem
  Va : PMIOPort  Port=1  Side=Left
  Vb : PMIOPort  Port=2  Side=Left
  Vc : PMIOPort  Port=3  Side=Left
  n : PMIOPort  Port=4  Side=Left
  Vabc : Outport  InitialOutput=0
  vabc(t) : Outport  Port=2  InitialOutput=0
  wires:
  Voltage  Measurement/1(V) -> Mux/1
  Voltage  Measurement1/1(V) -> Mux/2
  Voltage  Measurement2/1(V) -> Mux/3
  Voltage  Measurement/2(v(t)) -> Mux1/1
  Voltage  Measurement1/2(v(t)) -> Mux1/2
  Voltage  Measurement2/2(v(t)) -> Mux1/3
  Mux1/1 -> vabc(t)/1
  Mux/1 -> Vabc/1
  connections:
  Va/RConn1 -- Voltage  Measurement/LConn1
  Vb/RConn1 -- Voltage  Measurement1/LConn1
  Vc/RConn1 -- Voltage  Measurement2/LConn1
  n/RConn1 -- Voltage  Measurement2/LConn2 -- Voltage  Measurement1/LConn2 -- Voltage  Measurement/LConn2

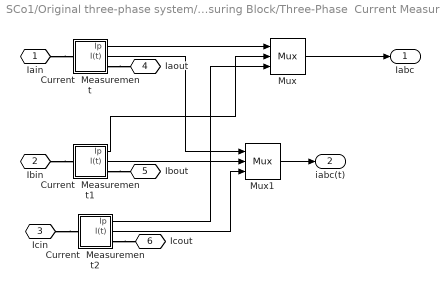
== system SCo1/Original three-phase system/Measuring Block/Three-Phase  Current Measurements ==
  Current  Measurement : Subsystem
  Current  Measurement1 : Subsystem
  Current  Measurement2 : Subsystem
  Mux : Mux  Inputs=3
  Mux1 : Mux  Inputs=3
  Iain : PMIOPort  Port=1  Side=Left
  Ibin : PMIOPort  Port=2  Side=Left
  Icin : PMIOPort  Port=3  Side=Left
  Iaout : PMIOPort  Port=4  Side=Right
  Ibout : PMIOPort  Port=5  Side=Right
  Icout : PMIOPort  Port=6  Side=Right
  Iabc : Outport  InitialOutput=0
  iabc(t) : Outport  Port=2  InitialOutput=0
  wires:
  Current  Measurement/1(Ip) -> Mux/1
  Current  Measurement1/1(Ip) -> Mux/2
  Current  Measurement2/1(Ip) -> Mux/3
  Mux1/1 -> iabc(t)/1
  Current  Measurement/2(I(t)) -> Mux1/1
  Current  Measurement1/2(I(t)) -> Mux1/2
  Current  Measurement2/2(I(t)) -> Mux1/3
  Mux/1 -> Iabc/1
  connections:
  Iain/RConn1 -- Current  Measurement/LConn1
  Current  Measurement/RConn1 -- Iaout/RConn1
  Ibin/RConn1 -- Current  Measurement1/LConn1
  Current  Measurement1/RConn1 -- Ibout/RConn1
  Icin/RConn1 -- Current  Measurement2/LConn1
  Current  Measurement2/RConn1 -- Icout/RConn1

== system SCo1/Analysis/Network with source decomposed in  symmetrical components/Load Voltage Measurements/Voltage  Measurement ==
  Fourier2 : powerlib_extras/Measurements/Fourier  f1=60  n=1
  Mux3 : Mux  Inputs=2
  Voltage Measurement1 : powerlib/Measurements/Voltage Measurement  PhasorSimulation=off  OutputType=Magnitude  PSBequivalent=0
  + : PMIOPort  Port=1  Side=Left
  - : PMIOPort  Port=2  Side=Left
  V : Outport  InitialOutput=0
  wires:
  Fourier2/1 -> Mux3/1
  Fourier2/2 -> Mux3/2
  Mux3/1 -> V/1
  Voltage Measurement1/1 -> Fourier2/1
  connections:
  +/RConn1 -- Voltage Measurement1/LConn1
  -/RConn1 -- Voltage Measurement1/LConn2

== system SCo1/Analysis/Network with source decomposed in  symmetrical components/Load Voltage Measurements/Voltage  Measurement1 ==
  Fourier2 : powerlib_extras/Measurements/Fourier  f1=60  n=1
  Mux3 : Mux  Inputs=2
  Voltage Measurement1 : powerlib/Measurements/Voltage Measurement  PhasorSimulation=off  OutputType=Magnitude  PSBequivalent=0
  + : PMIOPort  Port=1  Side=Left
  - : PMIOPort  Port=2  Side=Left
  V : Outport  InitialOutput=0
  wires:
  Mux3/1 -> V/1
  Fourier2/2 -> Mux3/2
  Fourier2/1 -> Mux3/1
  Voltage Measurement1/1 -> Fourier2/1
  connections:
  -/RConn1 -- Voltage Measurement1/LConn2
  +/RConn1 -- Voltage Measurement1/LConn1

== system SCo1/Analysis/Network with source decomposed in  symmetrical components/Load Voltage Measurements/Voltage  Measurement2 ==
  Fourier2 : powerlib_extras/Measurements/Fourier  f1=60  n=1
  Mux3 : Mux  Inputs=2
  Voltage Measurement1 : powerlib/Measurements/Voltage Measurement  PhasorSimulation=off  OutputType=Magnitude  PSBequivalent=0
  + : PMIOPort  Port=1  Side=Left
  - : PMIOPort  Port=2  Side=Left
  V : Outport  InitialOutput=0
  wires:
  Fourier2/1 -> Mux3/1
  Fourier2/2 -> Mux3/2
  Mux3/1 -> V/1
  Voltage Measurement1/1 -> Fourier2/1
  connections:
  +/RConn1 -- Voltage Measurement1/LConn1
  -/RConn1 -- Voltage Measurement1/LConn2

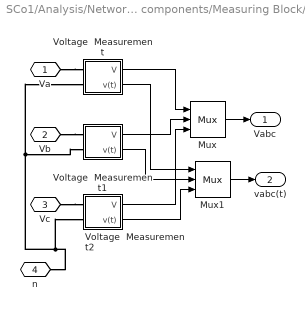
== system SCo1/Analysis/Network with source decomposed in  symmetrical components/Measuring Block/Three-Phase Voltage Measurements ==
  Mux : Mux  Inputs=3
  Mux1 : Mux  Inputs=3
  Voltage  Measurement : Subsystem
  Voltage  Measurement1 : Subsystem
  Voltage  Measurement2 : Subsystem
  Va : PMIOPort  Port=1  Side=Left
  Vb : PMIOPort  Port=2  Side=Left
  Vc : PMIOPort  Port=3  Side=Left
  n : PMIOPort  Port=4  Side=Left
  Vabc : Outport  InitialOutput=0
  vabc(t) : Outport  Port=2  InitialOutput=0
  wires:
  Voltage  Measurement/1(V) -> Mux/1
  Voltage  Measurement1/1(V) -> Mux/2
  Voltage  Measurement2/1(V) -> Mux/3
  Voltage  Measurement/2(v(t)) -> Mux1/1
  Voltage  Measurement1/2(v(t)) -> Mux1/2
  Voltage  Measurement2/2(v(t)) -> Mux1/3
  Mux1/1 -> vabc(t)/1
  Mux/1 -> Vabc/1
  connections:
  Va/RConn1 -- Voltage  Measurement/LConn1
  Vb/RConn1 -- Voltage  Measurement1/LConn1
  Vc/RConn1 -- Voltage  Measurement2/LConn1
  n/RConn1 -- Voltage  Measurement2/LConn2 -- Voltage  Measurement1/LConn2 -- Voltage  Measurement/LConn2

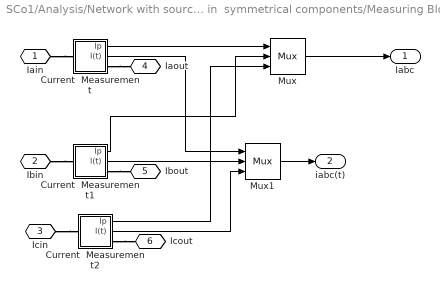
== system SCo1/Analysis/Network with source decomposed in  symmetrical components/Measuring Block/Three-Phase  Current Measurements ==
  Current  Measurement : Subsystem
  Current  Measurement1 : Subsystem
  Current  Measurement2 : Subsystem
  Mux : Mux  Inputs=3
  Mux1 : Mux  Inputs=3
  Iain : PMIOPort  Port=1  Side=Left
  Ibin : PMIOPort  Port=2  Side=Left
  Icin : PMIOPort  Port=3  Side=Left
  Iaout : PMIOPort  Port=4  Side=Right
  Ibout : PMIOPort  Port=5  Side=Right
  Icout : PMIOPort  Port=6  Side=Right
  Iabc : Outport  InitialOutput=0
  iabc(t) : Outport  Port=2  InitialOutput=0
  wires:
  Current  Measurement/1(Ip) -> Mux/1
  Current  Measurement1/1(Ip) -> Mux/2
  Current  Measurement2/1(Ip) -> Mux/3
  Mux1/1 -> iabc(t)/1
  Current  Measurement/2(I(t)) -> Mux1/1
  Current  Measurement1/2(I(t)) -> Mux1/2
  Current  Measurement2/2(I(t)) -> Mux1/3
  Mux/1 -> Iabc/1
  connections:
  Iain/RConn1 -- Current  Measurement/LConn1
  Current  Measurement/RConn1 -- Iaout/RConn1
  Ibin/RConn1 -- Current  Measurement1/LConn1
  Current  Measurement1/RConn1 -- Ibout/RConn1
  Icin/RConn1 -- Current  Measurement2/LConn1
  Current  Measurement2/RConn1 -- Icout/RConn1

== system SCo1/Original three-phase system/Measuring Block/Three-Phase Voltage Measurements/Voltage  Measurement ==
  Fourier2 : powerlib_extras/Measurements/Fourier  f1=60  n=1
  Mux3 : Mux  Inputs=2
  Voltage Measurement1 : powerlib/Measurements/Voltage Measurement  PhasorSimulation=off  OutputType=Magnitude  PSBequivalent=0
  + : PMIOPort  Port=1  Side=Left
  - : PMIOPort  Port=2  Side=Left
  V : Outport  InitialOutput=0
  v(t) : Outport  Port=2  InitialOutput=0
  wires:
  Fourier2/1 -> Mux3/1
  Fourier2/2 -> Mux3/2
  Mux3/1 -> V/1
  Voltage Measurement1/1 -> Fourier2/1, v(t)/1
  connections:
  +/RConn1 -- Voltage Measurement1/LConn1
  -/RConn1 -- Voltage Measurement1/LConn2

== system SCo1/Original three-phase system/Measuring Block/Three-Phase Voltage Measurements/Voltage  Measurement1 ==
  Fourier2 : powerlib_extras/Measurements/Fourier  f1=60  n=1
  Mux3 : Mux  Inputs=2
  Voltage Measurement1 : powerlib/Measurements/Voltage Measurement  PhasorSimulation=off  OutputType=Magnitude  PSBequivalent=0
  + : PMIOPort  Port=1  Side=Left
  - : PMIOPort  Port=2  Side=Left
  V : Outport  InitialOutput=0
  v(t) : Outport  Port=2  InitialOutput=0
  wires:
  Mux3/1 -> V/1
  Fourier2/2 -> Mux3/2
  Fourier2/1 -> Mux3/1
  Voltage Measurement1/1 -> v(t)/1, Fourier2/1
  connections:
  -/RConn1 -- Voltage Measurement1/LConn2
  +/RConn1 -- Voltage Measurement1/LConn1

== system SCo1/Original three-phase system/Measuring Block/Three-Phase Voltage Measurements/Voltage  Measurement2 ==
  Fourier2 : powerlib_extras/Measurements/Fourier  f1=60  n=1
  Mux3 : Mux  Inputs=2
  Voltage Measurement1 : powerlib/Measurements/Voltage Measurement  PhasorSimulation=off  OutputType=Magnitude  PSBequivalent=0
  + : PMIOPort  Port=1  Side=Left
  - : PMIOPort  Port=2  Side=Left
  V : Outport  InitialOutput=0
  v(t) : Outport  Port=2  InitialOutput=0
  wires:
  Fourier2/1 -> Mux3/1
  Fourier2/2 -> Mux3/2
  Mux3/1 -> V/1
  Voltage Measurement1/1 -> Fourier2/1, v(t)/1
  connections:
  +/RConn1 -- Voltage Measurement1/LConn1
  -/RConn1 -- Voltage Measurement1/LConn2

== system SCo1/Original three-phase system/Measuring Block/Three-Phase  Current Measurements/Current  Measurement ==
  Current Measurement1 : powerlib/Measurements/Current Measurement  PhasorSimulation=off  OutputType=Magnitude  PSBequivalent=0
  Fourier1 : powerlib_extras/Measurements/Fourier  f1=60  n=1
  Mux1 : Mux  Inputs=2
  + : PMIOPort  Port=1  Side=Left
  - : PMIOPort  Port=2  Side=Right
  Ip : Outport  InitialOutput=0
  I(t) : Outport  Port=2  InitialOutput=0
  wires:
  Fourier1/2 -> Mux1/2
  Fourier1/1 -> Mux1/1
  Mux1/1 -> Ip/1
  Current Measurement1/1 -> I(t)/1, Fourier1/1
  connections:
  +/RConn1 -- Current Measurement1/LConn1
  Current Measurement1/RConn1 -- -/RConn1

== system SCo1/Original three-phase system/Measuring Block/Three-Phase  Current Measurements/Current  Measurement1 ==
  Current Measurement1 : powerlib/Measurements/Current Measurement  PhasorSimulation=off  OutputType=Magnitude  PSBequivalent=0
  Fourier1 : powerlib_extras/Measurements/Fourier  f1=60  n=1
  Mux1 : Mux  Inputs=2
  + : PMIOPort  Port=1  Side=Left
  - : PMIOPort  Port=2  Side=Right
  Ip : Outport  InitialOutput=0
  I(t) : Outport  Port=2  InitialOutput=0
  wires:
  Mux1/1 -> Ip/1
  Fourier1/1 -> Mux1/1
  Fourier1/2 -> Mux1/2
  Current Measurement1/1 -> Fourier1/1, I(t)/1
  connections:
  Current Measurement1/RConn1 -- -/RConn1
  +/RConn1 -- Current Measurement1/LConn1

== system SCo1/Original three-phase system/Measuring Block/Three-Phase  Current Measurements/Current  Measurement2 ==
  Current Measurement1 : powerlib/Measurements/Current Measurement  PhasorSimulation=off  OutputType=Magnitude  PSBequivalent=0
  Fourier1 : powerlib_extras/Measurements/Fourier  f1=60  n=1
  Mux1 : Mux  Inputs=2
  + : PMIOPort  Port=1  Side=Left
  - : PMIOPort  Port=2  Side=Right
  Ip : Outport  InitialOutput=0
  I(t) : Outport  Port=2  InitialOutput=0
  wires:
  Fourier1/2 -> Mux1/2
  Fourier1/1 -> Mux1/1
  Mux1/1 -> Ip/1
  Current Measurement1/1 -> I(t)/1, Fourier1/1
  connections:
  +/RConn1 -- Current Measurement1/LConn1
  Current Measurement1/RConn1 -- -/RConn1

== system SCo1/Analysis/Network with source decomposed in  symmetrical components/Measuring Block/Three-Phase Voltage Measurements/Voltage  Measurement ==
  Fourier2 : powerlib_extras/Measurements/Fourier  f1=60  n=1
  Mux3 : Mux  Inputs=2
  Voltage Measurement1 : powerlib/Measurements/Voltage Measurement  PhasorSimulation=off  OutputType=Magnitude  PSBequivalent=0
  + : PMIOPort  Port=1  Side=Left
  - : PMIOPort  Port=2  Side=Left
  V : Outport  InitialOutput=0
  v(t) : Outport  Port=2  InitialOutput=0
  wires:
  Fourier2/1 -> Mux3/1
  Fourier2/2 -> Mux3/2
  Mux3/1 -> V/1
  Voltage Measurement1/1 -> Fourier2/1, v(t)/1
  connections:
  +/RConn1 -- Voltage Measurement1/LConn1
  -/RConn1 -- Voltage Measurement1/LConn2

== system SCo1/Analysis/Network with source decomposed in  symmetrical components/Measuring Block/Three-Phase Voltage Measurements/Voltage  Measurement1 ==
  Fourier2 : powerlib_extras/Measurements/Fourier  f1=60  n=1
  Mux3 : Mux  Inputs=2
  Voltage Measurement1 : powerlib/Measurements/Voltage Measurement  PhasorSimulation=off  OutputType=Magnitude  PSBequivalent=0
  + : PMIOPort  Port=1  Side=Left
  - : PMIOPort  Port=2  Side=Left
  V : Outport  InitialOutput=0
  v(t) : Outport  Port=2  InitialOutput=0
  wires:
  Mux3/1 -> V/1
  Fourier2/2 -> Mux3/2
  Fourier2/1 -> Mux3/1
  Voltage Measurement1/1 -> v(t)/1, Fourier2/1
  connections:
  -/RConn1 -- Voltage Measurement1/LConn2
  +/RConn1 -- Voltage Measurement1/LConn1

== system SCo1/Analysis/Network with source decomposed in  symmetrical components/Measuring Block/Three-Phase Voltage Measurements/Voltage  Measurement2 ==
  Fourier2 : powerlib_extras/Measurements/Fourier  f1=60  n=1
  Mux3 : Mux  Inputs=2
  Voltage Measurement1 : powerlib/Measurements/Voltage Measurement  PhasorSimulation=off  OutputType=Magnitude  PSBequivalent=0
  + : PMIOPort  Port=1  Side=Left
  - : PMIOPort  Port=2  Side=Left
  V : Outport  InitialOutput=0
  v(t) : Outport  Port=2  InitialOutput=0
  wires:
  Fourier2/1 -> Mux3/1
  Fourier2/2 -> Mux3/2
  Mux3/1 -> V/1
  Voltage Measurement1/1 -> Fourier2/1, v(t)/1
  connections:
  +/RConn1 -- Voltage Measurement1/LConn1
  -/RConn1 -- Voltage Measurement1/LConn2

== system SCo1/Analysis/Network with source decomposed in  symmetrical components/Measuring Block/Three-Phase  Current Measurements/Current  Measurement ==
  Current Measurement1 : powerlib/Measurements/Current Measurement  PhasorSimulation=off  OutputType=Magnitude  PSBequivalent=0
  Fourier1 : powerlib_extras/Measurements/Fourier  f1=60  n=1
  Mux1 : Mux  Inputs=2
  + : PMIOPort  Port=1  Side=Left
  - : PMIOPort  Port=2  Side=Right
  Ip : Outport  InitialOutput=0
  I(t) : Outport  Port=2  InitialOutput=0
  wires:
  Fourier1/2 -> Mux1/2
  Fourier1/1 -> Mux1/1
  Mux1/1 -> Ip/1
  Current Measurement1/1 -> I(t)/1, Fourier1/1
  connections:
  +/RConn1 -- Current Measurement1/LConn1
  Current Measurement1/RConn1 -- -/RConn1

== system SCo1/Analysis/Network with source decomposed in  symmetrical components/Measuring Block/Three-Phase  Current Measurements/Current  Measurement1 ==
  Current Measurement1 : powerlib/Measurements/Current Measurement  PhasorSimulation=off  OutputType=Magnitude  PSBequivalent=0
  Fourier1 : powerlib_extras/Measurements/Fourier  f1=60  n=1
  Mux1 : Mux  Inputs=2
  + : PMIOPort  Port=1  Side=Left
  - : PMIOPort  Port=2  Side=Right
  Ip : Outport  InitialOutput=0
  I(t) : Outport  Port=2  InitialOutput=0
  wires:
  Mux1/1 -> Ip/1
  Fourier1/1 -> Mux1/1
  Fourier1/2 -> Mux1/2
  Current Measurement1/1 -> Fourier1/1, I(t)/1
  connections:
  Current Measurement1/RConn1 -- -/RConn1
  +/RConn1 -- Current Measurement1/LConn1

== system SCo1/Analysis/Network with source decomposed in  symmetrical components/Measuring Block/Three-Phase  Current Measurements/Current  Measurement2 ==
  Current Measurement1 : powerlib/Measurements/Current Measurement  PhasorSimulation=off  OutputType=Magnitude  PSBequivalent=0
  Fourier1 : powerlib_extras/Measurements/Fourier  f1=60  n=1
  Mux1 : Mux  Inputs=2
  + : PMIOPort  Port=1  Side=Left
  - : PMIOPort  Port=2  Side=Right
  Ip : Outport  InitialOutput=0
  I(t) : Outport  Port=2  InitialOutput=0
  wires:
  Fourier1/2 -> Mux1/2
  Fourier1/1 -> Mux1/1
  Mux1/1 -> Ip/1
  Current Measurement1/1 -> I(t)/1, Fourier1/1
  connections:
  +/RConn1 -- Current Measurement1/LConn1
  Current Measurement1/RConn1 -- -/RConn1
